simulink library "Lib_HeatXfer_1DtransconductionCN_TMATS"  (R2019b)
settings: Solver=ode45  StartTime=0.0  StopTime=10.0  RelTol=1e-3  EnableMultiTasking=on
Description:
  | Thomas Modules
settings Model: Creator=jwchapm2  LastModifiedBy=bhisma
settings DataIOCC: LimitDataPoints=on  SaveFormat=Array  ReturnWorkspaceOutputs=off
settings OptimizationCC: ExpressionDepthLimit=2147483647  LifeSpan=inf
settings DebuggingCC: UnderspecifiedInitializationDetection=Classic  MergeDetectMultiDrivingBlocksExec=none  SolverPrmCheckMsg=warning  StateNameClashWarn=warning  SFUnexpectedBacktrackingDiag=warning  SFNoUnconditionalDefaultTransitionDiag=warning  SFExecutionAtInitializationDiag=none  ArithmeticOperatorsInVariantConditions=warning
settings HardwareCC: ProdBitPerPointer=32  ProdBitPerSizeT=32  ProdBitPerPtrDiffT=32  ProdLargestAtomicFloat=None  ProdIntDivRoundTo=Undefined  ProdEndianess=Unspecified  ProdWordSize=32  ProdHWDeviceType=32-bit Generic
settings ModelReferenceCC: PropagateSignalLabelsOutOfModel=off
settings SFSimCC: SimUseLocalCustomCode=off  CustomCodeUndefinedFunction=UseInterfaceOnly
settings RTWCC: RTWUseLocalCustomCode=off
settings CodeAppCC: StateflowObjectComments=on
settings GRTTargetCC: TargetLangStandard=C89/C90 (ANSI)  GeneratePreprocessorConditionals=Disable all
settings ConfigComp: CovMetricSettings=dw  CovHtmlReporting=on  CovSaveCumulativeToWorkspaceVar=on  CovSaveSingleToWorkspaceVar=on  CovExternalEMLEnable=off

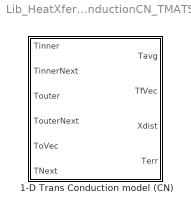
== system Lib_HeatXfer_1DtransconductionCN_TMATS ==
  1-D Trans Conduction model (CN) : Subsystem  mask(T-MATS: 1-D Trans Cond Model(CN) Block){dt_M=1, w_M=4, Nod_M=4, hB_M=1, kB_M=2, rhoB_M=3, cB_M=4, TypeA_M=off, wNodeA_M=1, hA_M=1, kA_M=2, rhoA_M=3, cA_M=4, TypeC_M=off, wNodeC_M=1, hC_M=1, kC_M=2, rhoC_M=3, cC_M=4}
      mask prompts: dt_M "dt_M - Time Step"; w_M "w_M - plate width"; Nod_M "Nod_M - number of plate nodes"; hB_M "hB_M - plate convection heat transfer coefficient"; kB_M "kB_M - plate thermal conductivity"; rhoB_M "rhoB_M - plate mass density"; cB_M "cB_M - plate specific heat"; TypeA_M "TypeA_M - Inner Barrier Material Type ( unset - fluid, set - solid)"; wNodeA_M "wNodeA_M - inner barrier node width"; hA_M "hA_M - convection heat transfer coefficient"; kA_M "kA_M - thermal conductivity"; rhoA_M "rhoA_M - mass density"; cA_M "cA_M - specific heat"; TypeC_M "TypeC_M - Outer Barrier Material Type ( unset - fluid, set - solid)"; wNodeC_M "wNodeC_M - outer barrier node width"; hC_M "hC_M - convection heat transfer coefficient"; kC_M "kC_M - thermal conductivity"; rhoC_M "rhoC_ M - mass density"; cC_M "cC_M - specific heat"
      mask help:
      | This function models the transient conduction of a plate (material B) with a fluid or a solid on either side (sides A and C) via the finite difference method (Crank-Nicolson).
      |
      | Setup requires the use of an external solver for determining Next temperature states. These Next temperatures are used to calcualte the current temperature. Calculated current temperature and the input current temperature are compared to generate the temperature error term used for convergence. It should be noted that TinnerNext and TouterNext/Tinner and Touter are defined as either the next and current (respectively) temperatures of the adjacent nodes or the gas temperatures depending on the application. (Press help button for more details)
      |
      | Export values are calculated based on a single time step. If additional dynamic behavior is required a simulink memory block may be used to update the temperature initial conditions.
      mask Help: web(which('HeatXfer_TMATS_1DTCondCN.html'),'-helpbrowser')
      mask Callback TypeA_M: MSK_SEC_Enables_TMATS('TypeA_M',[ 9 10 11 12 13],'en')
      mask Callback TypeC_M: MSK_SEC_Enables_TMATS('TypeC_M',[ 15 16 17 18 19],'en')
      mask DialogControl Container6_copy_copy Prompt: General
      mask DialogControl Container6 Prompt: Inner Material
      mask DialogControl Container6_copy Prompt: Outer Material

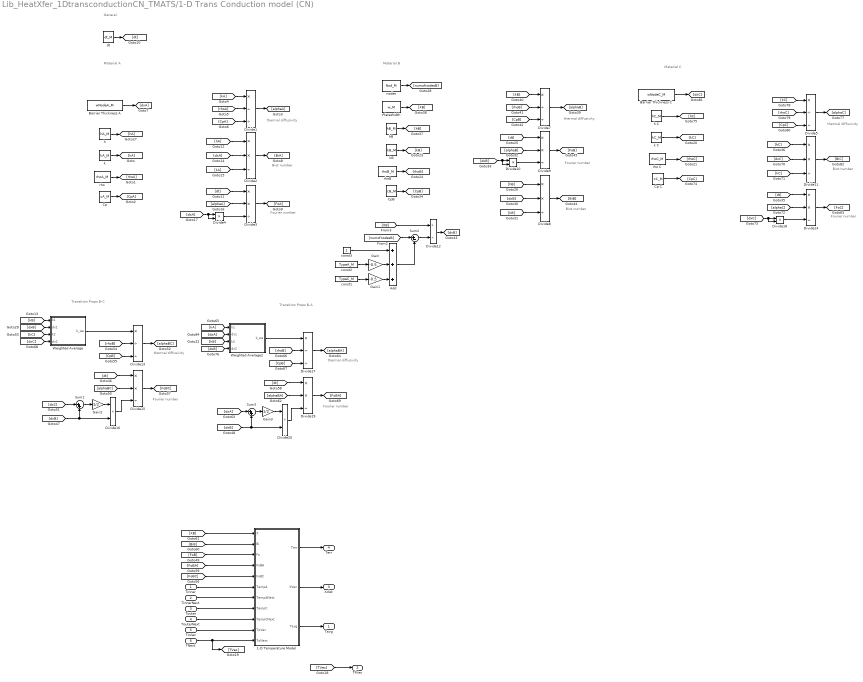
== system Lib_HeatXfer_1DtransconductionCN_TMATS/1-D Trans Conduction model (CN) ==
  note: Biot number
  note: Fourier number
  note: Fourier number
  note: Fourier number
  note: thermal diffusivity
  note: thermal diffusivity
  note: thermal diffusivity
  note: Transition Props B-A
  note: Transition Props B-C
  note: Material B
  note: Material A
  note: General
  note: thermal diffusivity
  note: Fourier number
  note: Biot number
  note: Fourier number
  note: Material C
  note: thermal diffusivity
  note: Biot number
  Tinner : Inport
  TinnerNext : Inport  Port=2
  Touter : Inport  Port=3
  TouterNext : Inport  Port=4
  ToVec : Inport  Port=5
  TNext : Inport  Port=6
  1-D Temperature Model : MATLAB Function  TreatAsAtomicUnit=on
  Add : Sum  Inputs=+++
  Barrier Thickness A : Constant  Value=wNodeA_M
  Barrier Thickness C : Constant  Value=wNodeC_M
  Cp : Constant  Value=cA_M
  Cp C : Constant  Value=cC_M
  CpB : Constant  Value=cB_M
  Divide{1,5,7,13,17} (5 alike) : Product  Inputs=*//
  Divide{4,10,16,18,20} (5 alike) : Product  Inputs=**
  Divide{2..3,8..9,11,14..15,19} (8 alike) : Product  Inputs=**/
  Divide12 : Product  Inputs=*/
  Gain : Gain  Gain=-0.5
  Gain1 : Gain  Gain=-0.5
  Gain2 : Gain  Gain=1/2
  Gain3 : Gain  Gain=1/2
  PlateWidth : Constant  Value=w_M
  Sum1 : Sum  Inputs=|++
  Sum2 : Sum  Inputs=|+-
  Sum3 : Sum  Inputs=|++
  Weighted Average : Subsystem
  Weighted Average2 : Subsystem
  const1 : Constant  Value=TypeC_M
  const2 : Constant  Value=TypeA_M
  const3 : Constant
  dt : Constant  Value=dt_M
  h : Constant  Value=hA_M
  h C : Constant  Value=hC_M
  hB : Constant  Value=hB_M
  k : Constant  Value=kA_M
  k C : Constant  Value=kC_M
  kB : Constant  Value=kB_M
  nodes : Constant  Value=Nod_M
  rho : Constant  Value=rhoA_M
  rho C : Constant  Value=rhoC_M
  rhoB : Constant  Value=rhoB_M
  Tavg : Outport
  TfVec : Outport  Port=2
  Xdist : Outport  Port=3
  Terr : Outport  Port=4
  wires:
  1-D Temperature Model/2(XVec) -> Xdist/1
  [BiB] -> 1-D Temperature Model/2(Bi)
  [dxB] -> Sum3/2, Divide20/2
  [dxB] -> Divide16/2, Sum1/2
  [CpB] -> Divide17/3
  [rhoB] -> Divide17/2
  Divide20/1 -> Divide19/3
  Divide17/1 -> [alphaBA]
  Divide19/1 -> [FoBA]
  [dxA] -> Sum3/1
  [alphaBA] -> Divide19/2
  [dt] -> Divide19/1
  [CpB] -> Divide13/3
  [rhoB] -> Divide13/2
  Divide16/1 -> Divide15/3
  Divide13/1 -> [alphaBC]
  Divide15/1 -> [FoBC]
  [dxC] -> Sum1/1
  [alphaBC] -> Divide15/2
  [dt] -> Divide15/1
  [CpB] -> Divide7/3
  [rhoB] -> Divide7/2
  Divide10/1 -> Divide9/3
  [hB] -> Divide8/1
  kB/1 -> [kB]
  rhoB/1 -> [rhoB]
  CpB/1 -> [CpB]
  Divide7/1 -> [alphaB]
  Divide8/1 -> [BiB]
  [kB] -> Divide8/3
  Divide9/1 -> [FoB]
  [kB] -> Divide7/1
  [dxB] -> Divide8/2
  nodes/1 -> [numofnodesB]
  [dxB] -> Divide10/2, Divide10/1
  [alphaB] -> Divide9/2
  [dt] -> Divide9/1
  hB/1 -> [hB]
  PlateWidth/1 -> [XB]
  [numofnodesB] -> Sum2/1
  const3/1 -> Add/1
  Sum2/1 -> Divide12/2
  [XB] -> Divide12/1
  Divide12/1 -> [dxB]
  [CpA] -> Divide1/3
  [rhoA] -> Divide1/2
  Divide4/1 -> Divide3/3
  [hA] -> Divide2/1
  k/1 -> [kA]
  rho/1 -> [rhoA]
  [FoB] -> 1-D Temperature Model/3(Fo)
  Cp/1 -> [CpA]
  Divide1/1 -> [alphaA]
  Divide2/1 -> [BiA]
  [kA] -> Divide2/3
  Divide3/1 -> [FoA]
  [kA] -> Divide1/1
  [dxA] -> Divide2/2
  [dxA] -> Divide4/1, Divide4/2
  dt/1 -> [dt]
  [alphaA] -> Divide3/2
  [dt] -> Divide3/1
  h/1 -> [hA]
  1-D Temperature Model/1(Terr) -> Terr/1
  ToVec/1 -> 1-D Temperature Model/10(ToVec)
  TinnerNext/1 -> 1-D Temperature Model/7(TempANext)
  TouterNext/1 -> 1-D Temperature Model/9(TempCNext)
  [CpC] -> Divide5/3
  [rhoC] -> Divide5/2
  Divide18/1 -> Divide14/3
  [hC] -> Divide11/1
  k C/1 -> [kC]
  rho C/1 -> [rhoC]
  Cp C/1 -> [CpC]
  Divide5/1 -> [alphaC]
  Divide11/1 -> [BiC]
  [kC] -> Divide11/3
  Divide14/1 -> [FoC]
  [kC] -> Divide5/1
  [dxC] -> Divide11/2
  Barrier Thickness C/1 -> [dxC]
  [dxC] -> Divide18/1, Divide18/2
  [alphaC] -> Divide14/2
  [dt] -> Divide14/1
  h C/1 -> [hC]
  Barrier Thickness A/1 -> [dxA]
  [XB] -> 1-D Temperature Model/1(X)
  [FoBA] -> 1-D Temperature Model/4(FoBA)
  [FoBC] -> 1-D Temperature Model/5(FoBC)
  1-D Temperature Model/3(Tavg) -> Tavg/1
  [TVec] -> TfVec/1
  TNext/1 -> [TVec], 1-D Temperature Model/11(ToNext)
  const2/1 -> Gain/1
  Gain/1 -> Add/2
  Gain1/1 -> Add/3
  const1/1 -> Gain1/1
  Add/1 -> Sum2/2
  Gain2/1 -> Divide16/1
  Sum1/1 -> Gain2/1
  Sum3/1 -> Gain3/1
  Gain3/1 -> Divide20/1
  Weighted Average2/1(k_wa) -> Divide17/1
  Tinner/1 -> 1-D Temperature Model/6(TempA)
  Touter/1 -> 1-D Temperature Model/8(TempC)
  [kB] -> Weighted Average/1(k1)
  [dxB] -> Weighted Average/2(dx1)
  [kC] -> Weighted Average/3(k2)
  [dxC] -> Weighted Average/4(dx2)
  Weighted Average/1(k_wa) -> Divide13/1
  [dxA] -> Weighted Average2/2(dx1)
  [dxB] -> Weighted Average2/4(dx2)
  [kA] -> Weighted Average2/1(k1)
  [kB] -> Weighted Average2/3(k2)

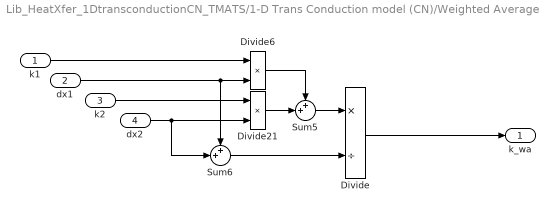
== system Lib_HeatXfer_1DtransconductionCN_TMATS/1-D Trans Conduction model (CN)/Weighted Average ==
  k1 : Inport
  dx1 : Inport  Port=2
  k2 : Inport  Port=3
  dx2 : Inport  Port=4
  Divide : Product  Inputs=*/
  Divide21 : Product  Inputs=**
  Divide6 : Product  Inputs=**
  Sum5 : Sum  Inputs=++|
  Sum6 : Sum  Inputs=++|
  k_wa : Outport
  wires:
  dx2/1 -> Sum6/2, Divide21/2
  dx1/1 -> Sum6/1, Divide6/2
  Divide21/1 -> Sum5/2
  Divide6/1 -> Sum5/1
  Divide/1 -> k_wa/1
  k2/1 -> Divide21/1
  Sum5/1 -> Divide/1
  k1/1 -> Divide6/1
  Sum6/1 -> Divide/2

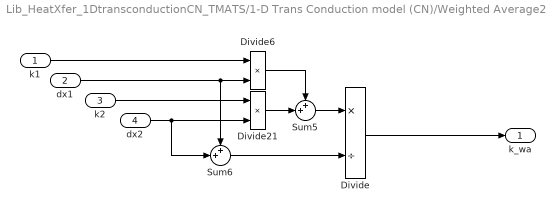
== system Lib_HeatXfer_1DtransconductionCN_TMATS/1-D Trans Conduction model (CN)/Weighted Average2 ==
  k1 : Inport
  dx1 : Inport  Port=2
  k2 : Inport  Port=3
  dx2 : Inport  Port=4
  Divide : Product  Inputs=*/
  Divide21 : Product  Inputs=**
  Divide6 : Product  Inputs=**
  Sum5 : Sum  Inputs=++|
  Sum6 : Sum  Inputs=++|
  k_wa : Outport
  wires:
  Sum6/1 -> Divide/2
  k1/1 -> Divide6/1
  Sum5/1 -> Divide/1
  k2/1 -> Divide21/1
  Divide/1 -> k_wa/1
  Divide6/1 -> Sum5/1
  Divide21/1 -> Sum5/2
  dx1/1 -> Divide6/2, Sum6/1
  dx2/1 -> Divide21/2, Sum6/2

== matlab function Lib_HeatXfer_1DtransconductionCN_TMATS/1-D Trans Conduction model (CN)/1-D Temperature Model ==
  data: X input; Bi input; Fo input; FoBA input; Terr output; XVec output; FoBC input; TempA input; TempANext input; TempC input; TempCNext input; ToVec input; ToNext input; Nod_M parameter; TypeA_M parameter; TypeC_M parameter; Tavg output
function [Terr, XVec,Tavg] = fcn(X, Bi, Fo, FoBA, FoBC, TempA,TempANext, TempC, TempCNext, ToVec,ToNext, Nod_M, TypeA_M, TypeC_M)
% This function models the heat transfer of a plate with fluid or material on either side
% on either side via the finite difference method (implicit),
% Per "Fundamentals of Heat and Mass Transfer" 5th edition, Incropera and
% DeWitt, section 5.9
%               |              |
%               |              |
%      Fluid    |    Solid B   |   Fluid
%        or     |              |    or   
%      Solid    |              |   Solid
%        A      |              |     C      
%               |              |         
% Inputs
% X - width of plate B
% Fo - Fourier number B = alpha * delta_t/ (delta_x)^2
% Bi - Biot number B = h * delta_x/k
% FoBA - Fourier number (in material B conduction from material A) = alpha * delta_t/ (delta_x)^2
% FoBC - Fourier number (in material B conduction from material C) = alpha * delta_t/ (delta_x)^2
% TempA - Inner barrier temperature 
% TempC - outer barrier temperature
% ToVec - current temperature states
% ToNext - next temperature states
% Nod_M - number of nodes for Solid B - 1 (located within the Mask)
% TypeA - Material A type (0 - fluid, 1 - solid, located within the Mask)
% TypeC - Material B type (0 - fluid, 1 - solid, located within the Mask)
%
% Outputs
% XVec - vector of distances from inner -> outer 
% Terr - Calculated temperature error vector

%Initialize
States = Nod_M;
XVec = zeros(States,1);
Nw = XVec;
ToCalc = ToVec;
dx = X/(States - (1 - 0.5*(TypeA_M + TypeC_M)));

% Calculate each updated node state

%Determine barrier A node temperature
if TypeA_M == 1 % barrier A is a solid (1) or fluid (other)
    Fwd = -(Fo*ToVec(2) + FoBA * TempA) + (Fo + FoBA)* ToVec(1);
    Back = -(Fo*ToNext(2) + FoBA * TempANext) + (Fo + FoBA)* ToNext(1);
    ToCalc(1) = 0.5*(Fwd+Back) + ToNext(1);
    XVec(1) = dx/2;
    Nw(1) = dx;
else
    Fwd = (2*Fo + 2*Bi*Fo)* ToVec(1) - 2*Fo*(ToVec(2) + Bi*TempA);
    Back = (2*Fo + 2*Bi*Fo)* ToNext(1) - 2*Fo*(ToNext(2) + Bi*TempANext);
    ToCalc(1) = 0.5*(Fwd+Back) + ToNext(1);
    XVec(1) = 0;
    Nw(1) = dx/2;
end


% Determine temperature of internal nodes
for i = 2: States -1
    Fwd = (2*Fo)*ToVec(i) - Fo * (ToVec(i+1) + ToVec(i-1));
    Back = (2*Fo)*ToNext(i) - Fo * (ToNext(i+1) + ToNext(i-1));
    ToCalc(i) = 0.5*(Fwd+Back) +  ToNext(i);
    XVec(i) = XVec(i-1) + dx;
    Nw(i) = dx;
end

%Determine barrier C node temperature
if TypeC_M == 1 % barrier C is a solid (1) or fluid (other)
    Fwd = -(Fo*ToVec(States - 1) + FoBC * TempC) + (Fo + FoBC)* ToVec(States);
    Back = -(Fo*ToNext(States - 1) + FoBC * TempCNext) + (Fo + FoBC)* ToNext(States);
    ToCalc(States) = 0.5*(Fwd+Back) +  ToNext(States);
    XVec(States) = XVec(States -1) + dx;
    Nw(States) = dx;
else
    Fwd = (2*Fo + 2*Bi*Fo)* ToVec(States) - 2*Fo*(ToVec(States - 1) + Bi*TempC);
    Back = (2*Fo + 2*Bi*Fo)* ToNext(States) - 2*Fo*(ToNext(States - 1) + Bi*TempCNext);
    ToCalc(States) = 0.5*(Fwd+Back) +  ToNext(States);
    XVec(States) = XVec(States -1) + dx;
    Nw(States) = dx/2;
end


%Determine error by comparing calculated Temperature with Actual
%temperature
Terr = (ToCalc - ToVec)./ToVec;
Tavg = sum(ToNext.*Nw)/sum(Nw);
